simulink model "SOHO_sim_v7"  (R2018b)
settings: Solver=ode113  StartTime=0.0  StopTime=3600  FixedStep=25  RelTol=1e-8  AbsTol=1e-10
undefined symbols (not defined in the file or in its folder): areas, att_det_method, bcs, DCM, I_vec, mu, mu1, normals, omega, r0, sc, v0, w0
libraries: aerolibnav x2, sharedutil x1
settings Model: Creator=ayotundedemuren  LastModifiedBy=Ethan
settings SolverCC: AutoScaleAbsTol=off

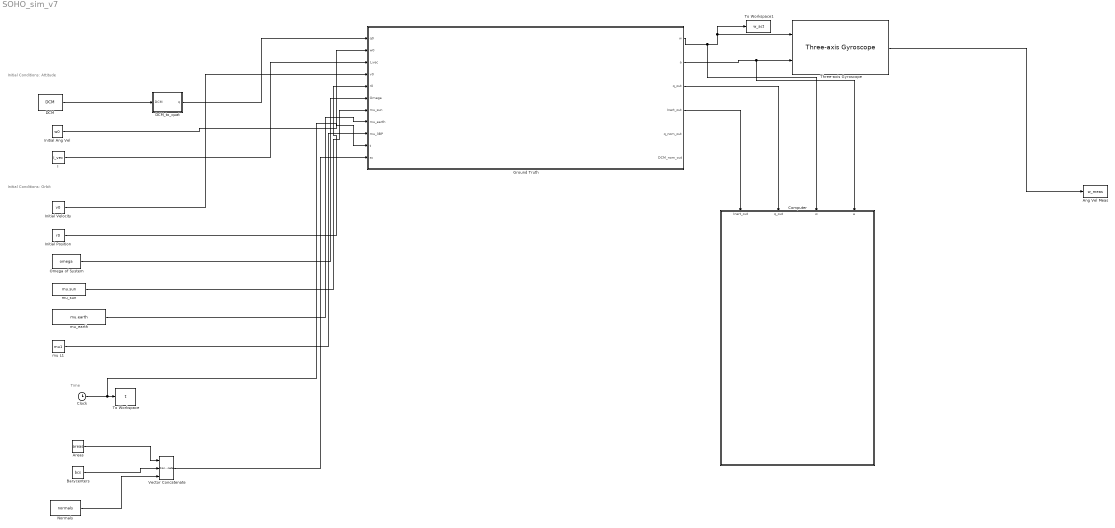
== system SOHO_sim_v7 ==
  note: Time
  note: Initial Conditions: Orbit
  note: Initial Conditions: Attitude
  Ang Vel Meas : ToWorkspace  VariableName=w_meas  SampleTime=-1
  Areas : Constant  Value=areas
  Barycenters : Constant  Value=bcs
  Clock : Clock
      settings: Decimation=100
  Computer : Subsystem
  DCM : Constant  Value=DCM
  DCM_to_quat : MATLAB Function  TreatAsAtomicUnit=on
  Ground Truth : Subsystem
  I : Constant  Value=I_vec
  Initial Ang Vel : Constant  Value=w0
  Initial Position : Constant  Value=r0
  Initial Velocity : Constant  Value=v0
  Normals : Constant  Value=normals
  Omega of System : Constant  Value=omega
  Three-axis Gyroscope : aerolibnav/Three-axis Gyroscope  dtype_g=on  w_g=190  z_g=0.707  g_sf_cc=[1 0 0; 0 1 0; 0 0 1]  g_bias=[0 0 0]  g_sen=[0 0 0]  g_Ts=0  g_rand=off  g_seeds=[23093 23094 23095]  g_pow=[0.0001 0.0001 0.0001]  g_sat="[-inf  -inf  -inf  inf inf inf]"
      settings: SourceProductName=Aerospace Blockset  SourceProductBaseCode=AE
  To Workspace : ToWorkspace  VariableName=t  SampleTime=-1
      settings: Save2DSignal=2-D array (concatenate along first dimension)
  To Workspace1 : ToWorkspace  VariableName=w_act  SampleTime=-1
  Vector Concatenate : Concatenate  NumInputs=3  Mode=Multidimensional array  ConcatenateDimension=2
  mu L1 : Constant  Value=mu1
  mu_earth : Constant  Value=mu.earth
  mu_sun : Constant  Value=mu.sun
  wires:
  Normals/1 -> Vector Concatenate/3
  Barycenters/1 -> Vector Concatenate/2
  Areas/1 -> Vector Concatenate/1
  Clock/1 -> Ground Truth/10(t), To Workspace/1
  DCM/1 -> DCM_to_quat/1(DCM)
  Three-axis Gyroscope/1 -> Ang Vel Meas/1
  DCM_to_quat/1(q) -> Ground Truth/1(q0)
  Initial Ang Vel/1 -> Ground Truth/2(w0)
  I/1 -> Ground Truth/3(I_vec)
  Initial Velocity/1 -> Ground Truth/4(v0)
  Initial Position/1 -> Ground Truth/5(r0)
  Omega of System/1 -> Ground Truth/6(Omega)
  mu_sun/1 -> Ground Truth/7(mu_sun)
  mu_earth/1 -> Ground Truth/8(mu_earth)
  mu L1/1 -> Ground Truth/9(mu_3BP)
  Vector Concatenate/1 -> Ground Truth/11(sc)
  Ground Truth/2(a) -> Computer/4(a), Three-axis Gyroscope/2
  Ground Truth/1(w) -> Computer/3(w), To Workspace1/1, Three-axis Gyroscope/1
  Ground Truth/3(q_out) -> Computer/2(q_out)
  Ground Truth/4(Inert_out) -> Computer/1(Inert_out)

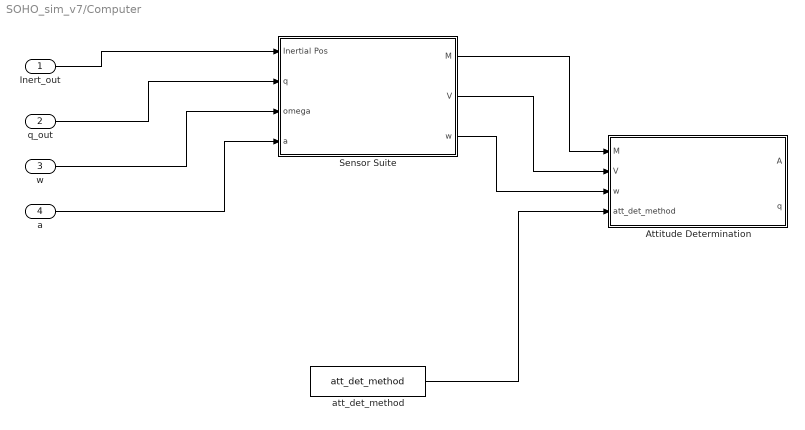
== system SOHO_sim_v7/Computer ==
  Inert_out : Inport
  q_out : Inport  Port=2
  w : Inport  Port=3
  a : Inport  Port=4
  Attitude Determination : MATLAB Function  TreatAsAtomicUnit=on
  Sensor Suite : Subsystem
  att_det_method : Constant  Value=att_det_method
  wires:
  Inert_out/1 -> Sensor Suite/1(Inertial Pos)
  q_out/1 -> Sensor Suite/2(q)
  Sensor Suite/1(M) -> Attitude Determination/1(M)
  Sensor Suite/2(V) -> Attitude Determination/2(V)
  att_det_method/1 -> Attitude Determination/4(att_det_method)
  Sensor Suite/3(w) -> Attitude Determination/3(w)
  w/1 -> Sensor Suite/3(omega)
  a/1 -> Sensor Suite/4(a)

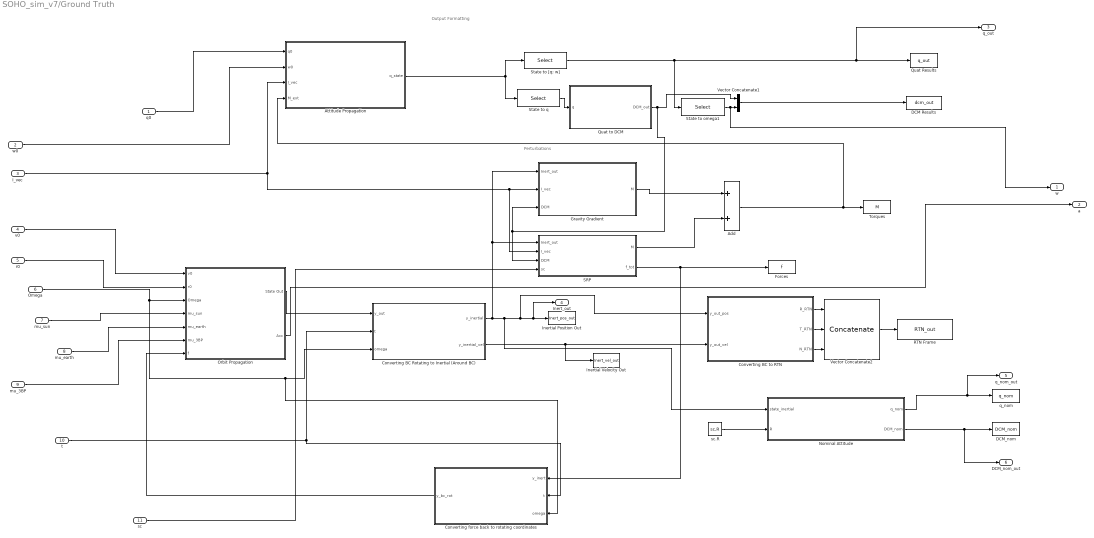
== system SOHO_sim_v7/Ground Truth ==
  note: Perturbations
  note: Output Formatting
  q0 : Inport
  w0 : Inport  Port=2
  I_vec : Inport  Port=3
  v0 : Inport  Port=4
  r0 : Inport  Port=5
  Omega : Inport  Port=6
  mu_sun : Inport  Port=7
  mu_earth : Inport  Port=8
  mu_3BP : Inport  Port=9
  t : Inport  Port=10
  sc : Inport  Port=11
  Add : Sum
  Attitude Propagation : Subsystem
  Converting BC Rotating to Inertial (Around BC) : MATLAB Function  TreatAsAtomicUnit=on
  Converting BC to RTN : MATLAB Function  TreatAsAtomicUnit=on
  Converting force back to rotating coordinates : MATLAB Function  TreatAsAtomicUnit=on
  DCM Results : ToWorkspace  VariableName=dcm_out  SampleTime=-1
      settings: Save2DSignal=2-D array (concatenate along first dimension)
  DCM_nom : ToWorkspace  VariableName=DCM_nom  SampleTime=-1
  Forces : ToWorkspace  VariableName=f  SampleTime=-1
  Gravity Gradient : MATLAB Function  TreatAsAtomicUnit=on
  Inertial Position Out : ToWorkspace  VariableName=Inert_pos_out  SampleTime=-1
  Inertial Velocity Out : ToWorkspace  VariableName=Inert_vel_out  SampleTime=-1
  Nominal Attitude : MATLAB Function  TreatAsAtomicUnit=on
  Orbit Propagation : Subsystem
  Quat Results : ToWorkspace  VariableName=q_out  SampleTime=-1
  Quat to DCM : MATLAB Function  TreatAsAtomicUnit=on
  RTN Frame : ToWorkspace  VariableName=RTN_out  SampleTime=-1
  SRP : MATLAB Function  TreatAsAtomicUnit=on
  State to [q; w] : Selector  InputPortWidth=10  IndexOptions=Starting index (dialog)  Indices=[1]  OutputSizes=7
  State to omega1 : Selector  InputPortWidth=7  IndexOptions=Starting index (dialog)  Indices=5  OutputSizes=3
  State to q : Selector  InputPortWidth=10  IndexOptions=Starting index (dialog)  Indices=[1]  OutputSizes=4
  Torques : ToWorkspace  VariableName=M  SampleTime=-1
  Vector Concatenate1 : Concatenate
  Vector Concatenate2 : Concatenate  NumInputs=3  Mode=Multidimensional array  ConcatenateDimension=2
  q_nom : ToWorkspace  VariableName=q_nom  SampleTime=-1
  sc.R : Constant  Value=sc.R
  w : Outport
  a : Outport  Port=2
  q_out : Outport  Port=3
  Inert_out : Outport  Port=4
  q_nom_out : Outport  Port=5
  DCM_nom_out : Outport  Port=6
  wires:
  Vector Concatenate2/1 -> RTN Frame/1
  State to [q; w]/1 -> State to omega1/1, q_out/1, Quat Results/1
  mu_sun/1 -> Orbit Propagation/4(mu_sun)
  Omega/1 -> Orbit Propagation/3(Omega), Converting force back to rotating coordinates/3(omega), Converting BC Rotating to Inertial (Around BC)/3(omega)
  Vector Concatenate1/1 -> DCM Results/1
  sc/1 -> SRP/4(sc)
  State to q/1 -> Quat to DCM/1(q)
  Quat to DCM/1(DCM_out) -> SRP/3(DCM), Gravity Gradient/3(DCM), Vector Concatenate1/1
  State to omega1/1 -> w/1, Vector Concatenate1/2
  r0/1 -> Orbit Propagation/2(r0)
  Nominal Attitude/1(q_nom) -> q_nom_out/1, q_nom/1
  I_vec/1 -> Attitude Propagation/3(I_vec), SRP/2(I_vec), Gravity Gradient/2(I_vec)
  Converting BC to RTN/1(R_RTN) -> Vector Concatenate2/1
  Add/1 -> Torques/1, Attitude Propagation/4(M_ext)
  SRP/2(f_tot) -> Converting force back to rotating coordinates/1(y_inert), Forces/1
  Orbit Propagation/1(State Out) -> Converting BC Rotating to Inertial (Around BC)/1(y_out)
  t/1 -> Converting BC Rotating to Inertial (Around BC)/2(t), Converting force back to rotating coordinates/2(t)
  Converting BC Rotating to Inertial (Around BC)/1(y_inertial) -> SRP/1(Inert_out), Gravity Gradient/1(Inert_out), Nominal Attitude/1(state_inertial), Converting BC to RTN/1(y_out_pos), Inert_out/1, Inertial Position Out/1
  Converting BC Rotating to Inertial (Around BC)/2(y_inertial_vel) -> Inertial Velocity Out/1, Converting BC to RTN/2(y_out_vel)
  q0/1 -> Attitude Propagation/1(q0)
  Converting BC to RTN/2(T_RTN) -> Vector Concatenate2/2
  Converting force back to rotating coordinates/1(y_bc_rot) -> Orbit Propagation/7(f)
  sc.R/1 -> Nominal Attitude/2(R)
  Nominal Attitude/2(DCM_nom) -> DCM_nom_out/1, DCM_nom/1
  v0/1 -> Orbit Propagation/1(v0)
  SRP/1(M) -> Add/2
  Attitude Propagation/1(q_state) -> State to [q; w]/1, State to q/1
  Gravity Gradient/1(M) -> Add/1
  Converting BC to RTN/3(N_RTN) -> Vector Concatenate2/3
  w0/1 -> Attitude Propagation/2(w0)
  mu_3BP/1 -> Orbit Propagation/6(mu_3BP)
  mu_earth/1 -> Orbit Propagation/5(mu_earth)
  Orbit Propagation/2(Acc) -> a/1

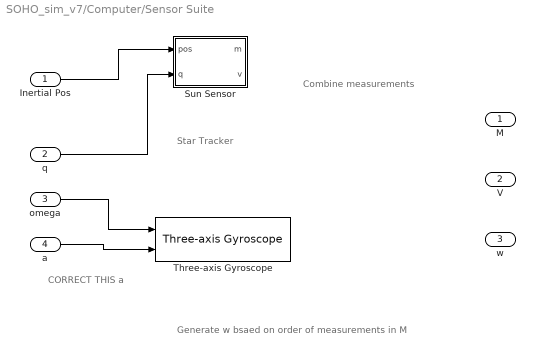
== system SOHO_sim_v7/Computer/Sensor Suite ==
  note: CORRECT THIS a
  note: Generate w bsaed on order of measurements in M
  note: Combine measurements
  note: Star Tracker
  Inertial Pos : Inport
  q : Inport  Port=2
  omega : Inport  Port=3
  a : Inport  Port=4
  Sun Sensor : MATLAB Function  TreatAsAtomicUnit=on
  Three-axis Gyroscope : aerolibnav/Three-axis Gyroscope  dtype_g=on  w_g=190  z_g=0.707  g_sf_cc=[1 0 0; 0 1 0; 0 0 1]  g_bias=[0 0 0]  g_sen=[0 0 0]  g_Ts=0  g_rand=on  g_seeds=[23093 23094 23095]  g_pow=[0.0001 0.0001 0.0001]  g_sat="[-inf  -inf  -inf  inf inf inf]"
      settings: SourceProductName=Aerospace Blockset  SourceProductBaseCode=AE
  M : Outport
  V : Outport  Port=2
  w : Outport  Port=3
  wires:
  Inertial Pos/1 -> Sun Sensor/1(pos)
  q/1 -> Sun Sensor/2(q)
  omega/1 -> Three-axis Gyroscope/1
  a/1 -> Three-axis Gyroscope/2

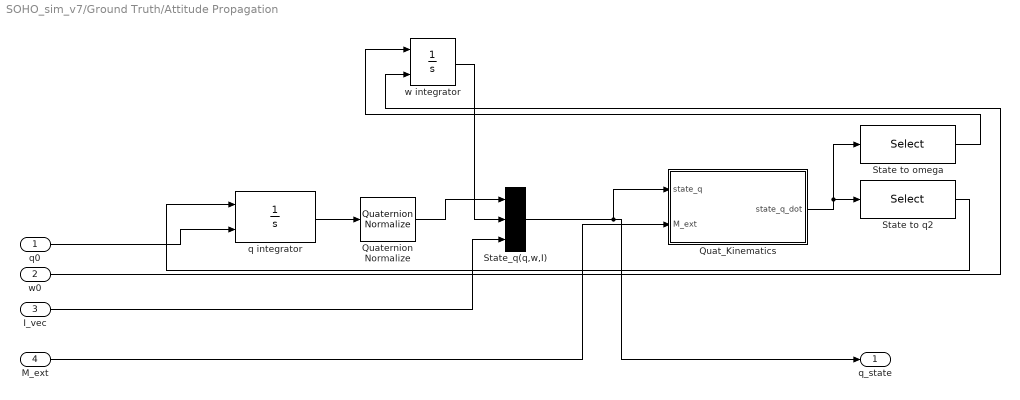
== system SOHO_sim_v7/Ground Truth/Attitude Propagation ==
  q0 : Inport
  w0 : Inport  Port=2
  I_vec : Inport  Port=3
  M_ext : Inport  Port=4
  Quat_Kinematics : MATLAB Function  TreatAsAtomicUnit=on
  Quaternion Normalize : sharedutil/Quaternion Normalize  aMode=aMode
      settings: SourceProductName=Aerospace Blockset  SourceProductBaseCode=AE
  State to omega : Selector  InputPortWidth=10  IndexOptions=Starting index (dialog)  Indices=5  OutputSizes=3
  State to q2 : Selector  InputPortWidth=10  IndexOptions=Starting index (dialog)  Indices=[1]  OutputSizes=4
  State_q(q,w,I) : Concatenate  NumInputs=3
  q integrator : Integrator  InitialConditionSource=external
  w integrator : Integrator  InitialConditionSource=external
  q_state : Outport
  wires:
  State_q(q,w,I)/1 -> q_state/1, Quat_Kinematics/1(state_q)
  w integrator/1 -> State_q(q,w,I)/2
  State to omega/1 -> w integrator/1
  Quat_Kinematics/1(state_q_dot) -> State to omega/1, State to q2/1
  State to q2/1 -> q integrator/1
  w0/1 -> w integrator/2
  q0/1 -> q integrator/2
  I_vec/1 -> State_q(q,w,I)/3
  M_ext/1 -> Quat_Kinematics/2(M_ext)
  Quaternion Normalize/1 -> State_q(q,w,I)/1
  q integrator/1 -> Quaternion Normalize/1

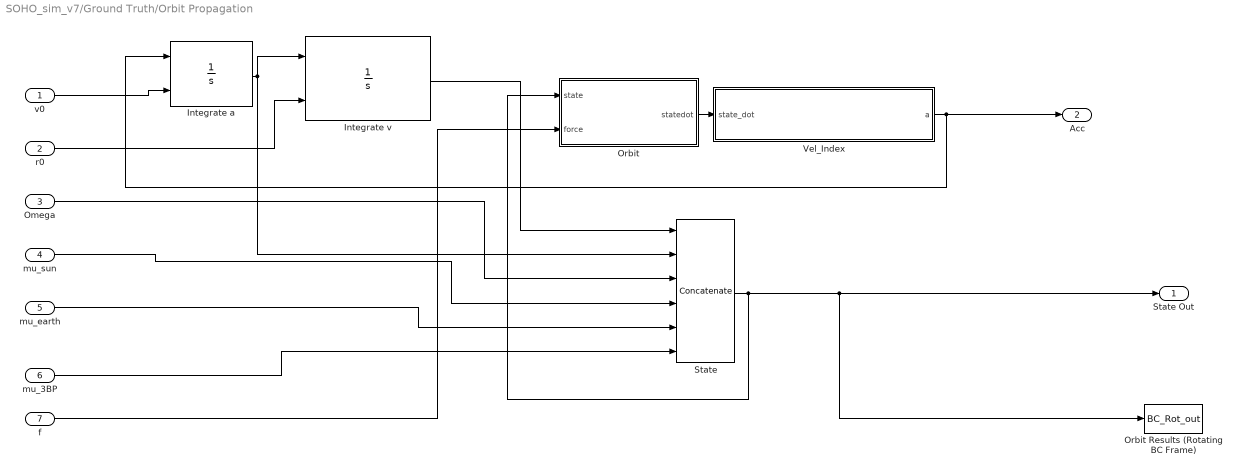
== system SOHO_sim_v7/Ground Truth/Orbit Propagation ==
  v0 : Inport
  r0 : Inport  Port=2
  Omega : Inport  Port=3
  mu_sun : Inport  Port=4
  mu_earth : Inport  Port=5
  mu_3BP : Inport  Port=6
  f : Inport  Port=7
  Integrate a : Integrator  InitialConditionSource=external  AbsoluteTolerance=1e-6
  Integrate v : Integrator  InitialConditionSource=external  AbsoluteTolerance=1e-6
  Orbit : MATLAB Function  TreatAsAtomicUnit=on
  Orbit Results (Rotating BC Frame) : ToWorkspace  VariableName=BC_Rot_out  SampleTime=-1
  "State " : Concatenate  NumInputs=6
  Vel_Index : MATLAB Function  TreatAsAtomicUnit=on
  State Out : Outport
  Acc : Outport  Port=2
  wires:
  r0/1 -> Integrate v/2
  Integrate a/1 -> "State "/2, Integrate v/1
  Integrate v/1 -> "State "/1
  "State "/1 -> Orbit/1(state), Orbit Results (Rotating BC Frame)/1, State Out/1
  Vel_Index/1(a) -> Integrate a/1, Acc/1
  Orbit/1(statedot) -> Vel_Index/1(state_dot)
  v0/1 -> Integrate a/2
  mu_3BP/1 -> "State "/6
  Omega/1 -> "State "/3
  mu_sun/1 -> "State "/4
  mu_earth/1 -> "State "/5
  f/1 -> Orbit/2(force)

== matlab function SOHO_sim_v7/Ground Truth/Orbit Propagation/Vel_Index ==
  data: state_dot input; a output
function a = fcn(state_dot)

a = state_dot(4:6);

end

== matlab function SOHO_sim_v7/Ground Truth/Orbit Propagation/Orbit ==
  data: state input; statedot output; force input
function statedot = fcn(state, force)
force = force*0;
dis_sun = 149599650;

statedot = zeros(length(state),1);
x = state(1);
y = state(2);
z = state(3);
xdot = state(4);
ydot = state(5);
zdot = state(6);

w = state(7);
mu1 = state(8);
mu2 = state(9);
mu_sys = state(10);

Rx1 = - mu_sys*dis_sun;
Rx2 = (1-mu_sys)*dis_sun;

R1 = sqrt((x - Rx1)^2 + y^2 + z^2);
R2 = sqrt((x - Rx2)^2 + y^2 + z^2);

statedot(1) = xdot;
statedot(2) = ydot;
statedot(3) = zdot;

statedot(4) = x*w^2 + 2*ydot*w + mu1 * (Rx1 - x)/R1^3 + mu2 * (Rx2 - x)/R2^3 + force(1);
statedot(5) = y*w^2 - 2*xdot*w - mu1 * (y)/R1^3 - mu2 * (y)/R2^3 + force(2);
statedot(6) = - mu1 * (z)/R1^3 - mu2 * (z)/R2^3 + force(3);
end

== matlab function SOHO_sim_v7/Ground Truth/Converting BC to RTN ==
  data: y_out_pos input; R_RTN output; T_RTN output; N_RTN output; y_out_vel input
function [R_RTN, T_RTN, N_RTN] = BCRot_to_RTN(y_out_pos, y_out_vel)
% 
% %% RTN Frame Rotating
% r = y_out(1:3);
% v = y_out(4:6);
% R_RTN = zeros(3,1);
% T_RTN = zeros(3,1);
% N_RTN = zeros(3,1);
% 
% for ii = 1:1
% 
%     R_RTN = r ./ norm(r);
%     N_RTN = cross(r,v) ./norm(cross(r,v));
%     T_RTN = cross(N_RTN, R_RTN) ./ norm(cross(N_RTN, R_RTN));
% end

%% RTN Frame Inertial
r = y_out_pos(1:3);
v = y_out_vel(1:3);
R_RTN = zeros(3,1);
T_RTN = zeros(3,1);
N_RTN = zeros(3,1);

for ii = 1:1

    R_RTN = r ./ norm(r);
    N_RTN = cross(r,v) ./norm(cross(r,v));
    T_RTN = cross(N_RTN, R_RTN) ./ norm(cross(N_RTN, R_RTN));
end
end

== matlab function SOHO_sim_v7/Ground Truth/Converting BC Rotating to Inertial (Around BC) ==
  data: y_out input; y_inertial output; t input; omega input; y_inertial_vel output
function [y_inertial, y_inertial_vel] = BCRot_to_Inertial(y_out, t, omega)
wt = omega * t;
R = zeros(3,3);
R(1,:) = [cos(wt) sin(wt) 0];
R(2,:) = [-sin(wt) cos(wt) 0];
R(3,:) = [0 0 1];

sun_init = [-4.548476597303452e+02; 0; 0];
earth_init = [1.495991951523403e+08; 0; 0];
y_inertial = zeros(9, 1);
y_inertial_vel = zeros(9, 1);

y_inertial(1:3) = R' * y_out(1:3);
y_inertial_vel(1:3) = R' * y_out(4:6) + cross([0; 0; omega], y_inertial(1:3));
y_inertial(4:6) = R' * sun_init;
y_inertial_vel(4:6) = cross([0; 0; omega], y_inertial(4:6));
y_inertial(7:9) = R' * earth_init;
y_inertial_vel(7:9) = cross([0; 0; omega], y_inertial(7:9));
end

== matlab function SOHO_sim_v7/Ground Truth/Attitude Propagation/Quat_Kinematics ==
  data: state_q input; state_q_dot output; M_ext input
function state_q_dot  = quat_kin(state_q, M_ext)
% state = [q1 q2 q3 q4 w1 w2 w3 I1 I2 I3]

state_q_dot = zeros(length(state_q),1);
wx = state_q(5);
wy = state_q(6);
wz = state_q(7);
%% Kinematic Equations
Omega = [0 wz -wy wx; -wz 0 wx wy; wy -wx 0 wz; -wx -wy -wz 0];
err = 1 - norm(state_q(1:4));
state_q_dot(1:4) = 1/2 * Omega * state_q(1:4) + 0.05 * err * state_q(1:4);

%% Euler Equations
state_q_dot(5:end) = euler_eq(state_q(5:end), M_ext);
% state_q_dot(5) = -wy*wz * (state_q(10) - state_q(9))/state_q(8);
% state_q_dot(6) = -wx*wz * (state_q(8) - state_q(10))/state_q(9);
% state_q_dot(7) = -wx*wy * (state_q(9) - state_q(8))/state_q(10);

end

== matlab function SOHO_sim_v7/DCM_to_quat ==
  data: DCM input; q output
function q  = DCM_to_quat(DCM)
B4 = 1/4 * (1 + trace(DCM));
B1 = 1/4 * (1 + 2*DCM(1,1) - trace(DCM));
B2 = 1/4 * (1 + 2*DCM(2,2) - trace(DCM));
B3 = 1/4 * (1 + 2*DCM(3,3) - trace(DCM));
B = [B1 B2 B3 B4];
[M, I] = max(B);
q = zeros(4,1);
% q(4) = sqrt(B(I));
q(I) = sqrt(B(I));
if I == 4
    q(1) = (DCM(2,3) - DCM(3,2)) / 4 / q(I);
    q(2) = (DCM(3,1) - DCM(1,3)) / 4 / q(I);
    q(3) = (DCM(1,2) - DCM(2,1)) / 4 / q(I);
elseif I == 3
%     q(2) = (DCM(2,3) + DCM(3,2)) / 4 / q(4);
%     q(1) = (DCM(3,1) + DCM(1,3)) / 4 / q(4);
%     q(3) = (DCM(1,2) - DCM(2,1)) / 4 / q(4);
    
    q(2) = (DCM(2,3) + DCM(3,2)) / 4 / q(I);
    q(1) = (DCM(3,1) + DCM(1,3)) / 4 / q(I);
    q(4) = (DCM(1,2) - DCM(2,1)) / 4 / q(I);
elseif I == 2
%     q(2) = (DCM(2,3) + DCM(3,2)) / 4 / q(4);
%     q(3) = (DCM(3,1) - DCM(1,3)) / 4 / q(4);
%     q(1) = (DCM(1,2) + DCM(2,1)) / 4 / q(4);
    q(3) = (DCM(2,3) + DCM(3,2)) / 4 / q(I);
    q(4) = (DCM(3,1) - DCM(1,3)) / 4 / q(I);
    q(1) = (DCM(1,2) + DCM(2,1)) / 4 / q(I);
elseif I == 1
%     q(3) = (DCM(2,3) - DCM(3,2)) / 4 / q(4);
%     q(2) = (DCM(3,1) + DCM(1,3)) / 4 / q(4);
%     q(1) = (DCM(1,2) + DCM(2,1)) / 4 / q(4);
    q(4) = (DCM(2,3) - DCM(3,2)) / 4 / q(I);
    q(3) = (DCM(3,1) + DCM(1,3)) / 4 / q(I);
    q(2) = (DCM(1,2) + DCM(2,1)) / 4 / q(I);
end
q = q/norm(q);
end

== matlab function SOHO_sim_v7/Ground Truth/Gravity Gradient ==
  data: Inert_out input; M output; I_vec input; DCM input
function M = grav_grad(Inert_out, I_vec, DCM)
% Inert_out = [sat; sun; earth]

x = Inert_out(1);
y = Inert_out(2);
z = Inert_out(3);

x_s = Inert_out(4);
y_s = Inert_out(5);
z_s = Inert_out(6);

x_e = Inert_out(7);
y_e = Inert_out(8);
z_e = Inert_out(9);

Ix_sat = I_vec(1);
Iy_sat = I_vec(2);
Iz_sat = I_vec(3);

R_s = sqrt(((x - x_s).^2)+((y - y_s).^2)+((z - z_s).^2));
R_e = sqrt(((x - x_e).^2)+((y - y_e).^2)+((z - z_e).^2));

[A] = out2mat(DCM);
c_vec_s = A * [x-x_s; y-y_s; z-z_s];
cx_s = c_vec_s(1)/R_s;
cy_s = c_vec_s(2)/R_s;
cz_s = c_vec_s(3)/R_s;

c_vec_e = A * [x-x_e; y-y_e; z-z_e];
cx_e = c_vec_e(1)/R_e;
cy_e = c_vec_e(2)/R_e;
cz_e = c_vec_e(3)/R_e;

mu_earth = 3.986004418000000e+05;
mu_sun =  1.327124400180000e+11;

M_earth = (3*mu_earth./(R_e.^3)).*[((Iz_sat - Iy_sat).*cy_e.*cz_e)';...
    ((Ix_sat - Iz_sat).*cz_e.*cx_e)';...
    ((Iy_sat - Ix_sat).*cx_e.*cy_e)'];

M_sun = (3*mu_sun./(R_s.^3)).*[((Iz_sat - Iy_sat).*cy_s.*cz_s)';...
    ((Ix_sat - Iz_sat).*cz_s.*cx_s)';...
    ((Iy_sat - Ix_sat).*cx_s.*cy_s)'];

M = M_earth + M_sun;

== matlab function SOHO_sim_v7/Ground Truth/Quat to DCM ==
  data: q input; DCM_out output
function DCM_out  = quat_to_DCM(q)

DCM = zeros(3, 3);
DCM(:, :) = ((q(4)^2 - norm(q(1:3))^2)*eye(3) ...
    + 2 * q(1:3) * q(1:3)'...
    - 2 * q(4) * ...
    [0, -q(3), q(2); q(3), 0, -q(1); ...
    -q(2), q(1), 0]);

DCM_out = DCM(:)';
end

== matlab function SOHO_sim_v7/Ground Truth/Converting force back to rotating coordinates ==
  data: y_inert input; y_bc_rot output; t input; omega input
function y_bc_rot  = Inertial_to_BCRot(y_inert, t, omega)
wt = omega * t;
R = zeros(3,3);
R(1,:) = [cos(wt) sin(wt) 0];
R(2,:) = [-sin(wt) cos(wt) 0];
R(3,:) = [0 0 1];

y_bc_rot = zeros(3, 1);

y_bc_rot(1:3) = R * y_inert(1:3);

end

== matlab function SOHO_sim_v7/Ground Truth/Nominal Attitude ==
  data: state_inertial input; q_nom output; DCM_nom output; R input
function [q_nom, DCM_nom] = nominal(state_inertial, R)
sat_pos = state_inertial(1:3);
sun_pos = state_inertial(4:6);

vect_to_sun = (sun_pos - sat_pos) / norm((sun_pos - sat_pos));
b_x = vect_to_sun;
b_y = cross([0; 0; 1], b_x);
b_z = cross(b_x, b_y);

DCM_nom_temp = R'*[b_x'; b_y'; b_z'];
q_nom = DCM_to_quat(DCM_nom_temp);

DCM_nom = DCM_nom_temp(:);


end

== matlab function SOHO_sim_v7/Computer/Attitude Determination ==
  data: M input; A output; V input; w input; att_det_method input; q output
function [A, q] = att_det(M, V, w, att_det_method)

if att_det_method == 0
    A = det_method(M, V);
    q = DCM_to_quat(A);
    
elseif att_det_method == 1
    W = zeros(3, length(w));
    V2 = zeros(3, length(w));
    for ii = 1:length(w)
        W(:, ii) = sqrt(w(ii)).*M(:, ii);
        V2(:, ii) = sqrt(w(ii)).*V(:, ii);
    end
    [A, q] = q_method(W, V2);
    
elseif att_det_method == 2
    A = eyes(3);
    q = ones(4,1);
end

end

== matlab function SOHO_sim_v7/Computer/Sensor Suite/Sun Sensor ==
  data: pos input; m output; q input; v output
function [m, v] = sun_sens(pos, q)
% Basic sun sensor

A = q_to_DCM(q);
v = (pos(4:6) - pos(1:3)) / norm((pos(4:6) - pos(1:3))); % sun to sat vec
m = A * v; % currently this will give the exact measurement back 

end

== matlab function SOHO_sim_v7/Ground Truth/SRP ==
  data: Inert_out input; M output; I_vec input; DCM input; sc input; f_tot output
function [M,f_tot] = SRP(Inert_out, I_vec, DCM,sc)

F = 1358; % solar constant
c = 3e8;
P = F/c;
% sc data
areas = sc(1:end,1);
bcs = sc(1:end,2:4);
normals = sc(1:end,5:7);
% Principal Moments of Inertia
Ix_sat = I_vec(1);
Iy_sat = I_vec(2);
Iz_sat = I_vec(3);
% Inertial Sat Coordinates
x = Inert_out(1);
y = Inert_out(2);
z = Inert_out(3);
% Inertial Sun Coordinates
x_s = Inert_out(4);
y_s = Inert_out(5);
z_s = Inert_out(6);
% DCM
[A] = out2mat(DCM);
% Relative Sun to Sat Vector

r_sat2s = [x_s-x,y_s-y,z_s-z]; % vector
R_s2s = sqrt((r_sat2s(1).^2)+(r_sat2s(2).^2)+(r_sat2s(3).^2)); % magnitude
r_sp = A*r_sat2s'; % sun vector in principal frame
r_sp_hat = r_sp./R_s2s;

% SRP Coefficients
C_a = 0.1;
C_s = 0.2;
C_d = 0.7;

% initialize
M = [0,0,0]';
f = [0,0,0]';
f_tot = zeros(3,1);
r_press = zeros(3,1);
s_hat = r_sp_hat;

% Calculate SRP Force and Moment
for i = 1:length(areas)
    bc = bcs(i,:);
    area = areas(i);
    normal = normals(i,:);
    r_press = bc';
    n_hat = normal';
%     theta = atan2d(norm(cross(s_hat,n_hat)),dot(s_hat,n_hat));
    theta = acosd(dot(s_hat,n_hat));
    if dot(n_hat,s_hat) > 0 
        f = -P * area * cosd(theta)*((1-C_s)*s_hat + 2*(C_s*cosd(theta)+1/3*C_d)*n_hat);
        f_tot = f_tot + f;
        M = M + cross(r_press,f);
    else
    end
end
